simulink model "sixstep"  (R2017b)
settings: Solver=FixedStepDiscrete  StartTime=0.0  StopTime=10.0  FixedStep=0.003  RelTol=1e-3
libraries: simulink x1
settings Model: Creator=EW  LastModifiedBy=EW
settings DataIOCC: LimitDataPoints=on  SaveFormat=Array
settings OptimizationCC: LifeSpan=1
settings DebuggingCC: SFUnexpectedBacktrackingDiag=warning  SFNoUnconditionalDefaultTransitionDiag=warning  SFExecutionAtInitializationDiag=none
settings HardwareCC: ProdBitPerPointer=32  ProdBitPerSizeT=32  ProdBitPerPtrDiffT=32  ProdLargestAtomicInteger=Long  ProdLargestAtomicFloat=Double  ProdIntDivRoundTo=Undefined  ProdWordSize=32  ProdHWDeviceType=ARM Compatible->ARM Cortex
settings ModelReferenceCC: PropagateSignalLabelsOutOfModel=off
settings SFSimCC: MATLABDynamicMemAlloc=off
settings RTWCC: SystemTargetFile=mbed.tlc  TemplateMakefile=mbed.tmf  Description=Mbed Target (Embedded Target)  TargetLang=C++
settings CodeAppCC: IgnoreCustomStorageClasses=off  StateflowObjectComments=on
settings STFCustomTargetCC: TargetLibSuffix=.a  GenerateSampleERTMain=on  CombineOutputUpdateFcns=on  ERTCustomFileBanners=on  SupportContinuousTime=off  SupportNonInlinedSFcns=off  RemoveResetFunc=on  MATLABClassNameForMDSCustomization=Simulink.SoftwareTarget.ERTCustomization  ModelStepFunctionPrototypeControlCompliant=on  GRTInterface=off  SystemTargetFile=mbed.tlc
settings ERTTargetCC: MultiwordLength=2048  GenerateSampleERTMain=on  ParMdlRefBuildCompliant=off  CompOptLevelCompliant=off  ConcurrentExecutionCompliant=off  CPPClassGenCompliant=off  UseToolchainInfoCompliant=off  ERTCustomFileTemplate=mbed_file_process.tlc  ConvertIfToSwitch=off  SuppressUnreachableDefaultCases=off
settings ConfigComp: CovMetricSettings=dw  CovHtmlReporting=on  CovSaveCumulativeToWorkspaceVar=on  CovSaveSingleToWorkspaceVar=on  CovExternalEMLEnable=off

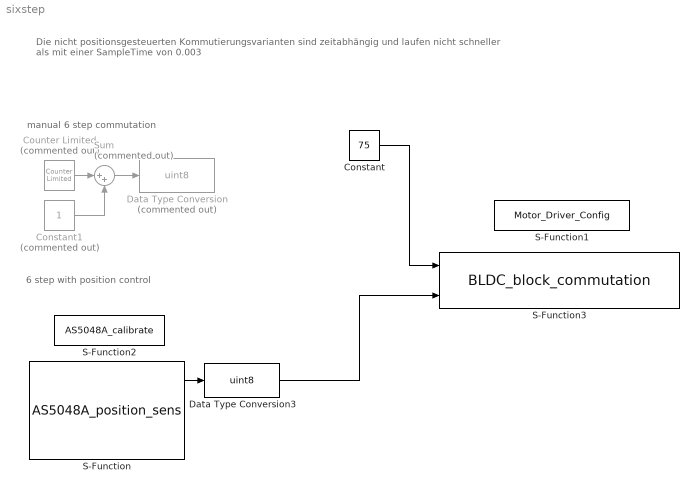
== system sixstep ==
  note: manual 6 step commutation
  note: 6 step with position control
  note: Die nicht positionsgesteuerten Kommutierungsvarianten sind zeitabhängig und laufen nicht schneller als mit einer SampleTime von 0.003
  Constant : Constant  Value=75  OutDataTypeStr=uint8
  Constant1 : Constant  Commented=on
  Counter Limited : simulink/Sources/Counter Limited  Commented=on  uplimit=5  tsamp=-1
  Data Type Conversion : DataTypeConversion  Commented=on  OutDataTypeStr=uint8
  Data Type Conversion3 : DataTypeConversion  OutDataTypeStr=uint8
  S-Function : S-Function  Priority=0  FunctionName=AS5048A_position_sens  Parameters=SampleTime, uint8(PortName), uint8(PinNumber)  SFunctionDeploymentMode=off  EnableBusSupport=off  mask{PortName=C, PinNumber=8, SampleTime=-1}
      mask prompts: PinNumber "Pin Number:"; SampleTime "Sample time (-1 for inherited)"
      mask TypeOptions PortName: A | B | C | D | F | G | H | I | J | K
      mask TypeOptions PinNumber: 0 | 1 | 2 | 3 | 4 | 5 | 6 | 7 | 8 | 9 | 10 | 11 | 12 | 13 | 14 | 15
      mask Display:
      | disp('AS5048')
      | port_label('output',1,'RAW');
      | port_label('output',2,'rad');
      | port_label('output',3,'rad/s');
  S-Function1 : S-Function  Priority=1  FunctionName=Motor_Driver_Config  Parameters=uint8(PWMUport),uint8(PWMVport),uint8(PWMWport),uint8(PWMUpin),uint8(PWMVpin),uint8(PWMWpin),uint8(EnableUport),uint8(EnableVport),uint8(EnableWport),uint8(EnableUpin),uint8(EnableVpin),uint8(EnableWpin)  SFunctionDeploymentMode=off  EnableBusSupport=off  mask{PWMUport=A, PWMUpin=8, PWMVport=A, PWMVpin=9, PWMWport=A, PWMWpin=10, EnableUport=C, EnableUpin=10, EnableVport=C, EnableVpin=11, EnableWport=C, EnableWpin=12}
      mask prompts: PWMUport "PWM   U:      Port Name"; PWMUpin "Pin Number"; PWMVport "PWM   V:      Port Name"; PWMVpin "Pin Number"; PWMWport "PWM  W:      Port Name"; PWMWpin "Pin Number"; EnableUport "Enable  U:     Port Name"; EnableUpin "Pin Number"; EnableVport "Enable  V:     Port Name"; EnableVpin "Pin Number"; EnableWport "Enable W:     Port Name"; EnableWpin "Pin Number"
      mask TypeOptions PWMUport: A | B | C | D | E | F | G | H | I | J
      mask TypeOptions PWMUpin: 0 | 1 | 2 | 3 | 4 | 5 | 6 | 7 | 8 | 9 | 10 | 11 | 12 | 13 | 14 | 15
      mask TypeOptions PWMVport: A | B | C | D | E | F | G | H | I | J
      mask TypeOptions PWMVpin: 0 | 1 | 2 | 3 | 4 | 5 | 6 | 7 | 8 | 9 | 10 | 11 | 12 | 13 | 14 | 15
      mask TypeOptions PWMWport: A | B | C | D | E | F | G | H | I | J
      mask TypeOptions PWMWpin: 0 | 1 | 2 | 3 | 4 | 5 | 6 | 7 | 8 | 9 | 10 | 11 | 12 | 13 | 14 | 15
      mask TypeOptions EnableUport: A | B | C | D | E | F | G | H | I | J
      mask TypeOptions EnableUpin: 0 | 1 | 2 | 3 | 4 | 5 | 6 | 7 | 8 | 9 | 10 | 11 | 12 | 13 | 14 | 15
      mask TypeOptions EnableVport: A | B | C | D | E | F | G | H | I | J
      mask TypeOptions EnableVpin: 0 | 1 | 2 | 3 | 4 | 5 | 6 | 7 | 8 | 9 | 10 | 11 | 12 | 13 | 14 | 15
      mask TypeOptions EnableWport: A | B | C | D | E | F | G | H | I | J
      mask TypeOptions EnableWpin: 0 | 1 | 2 | 3 | 4 | 5 | 6 | 7 | 8 | 9 | 10 | 11 | 12 | 13 | 14 | 15
  S-Function2 : S-Function  Priority=2  FunctionName=AS5048A_calibrate  SFunctionDeploymentMode=off  EnableBusSupport=off
      mask Display: disp('AS5048 calibration')
  S-Function3 : S-Function  Priority=3  FunctionName=BLDC_block_commutation  Parameters=SampleTime, uint8(power),uint8(mode)  SFunctionDeploymentMode=off  EnableBusSupport=off  mask{mode=Position controlled(AS5048A), power=on, SampleTime=-1}
      mask prompts: mode "chose operation mode"; power "Enable Power regulation port"; SampleTime "Sample time(-1 for inherited):"
      mask help:
      | power: is a pwm dutycycle in %   uses values 0-100
      |
      | step: provide the step sequence for the bldc driver uses values 1-6
      |
      | position: requires the position determined by the AS5048A_pos_sens Block
      mask TypeOptions mode: automatic steps | manual steps | Position controlled(AS5048A)
      mask Display:
      | disp(['6 Step Block Commutation'])
      | 
      | if power
      |     port_label('input',1,'power');
      | 
      |      if mode==2
      |         port_label('input',2,'step');
      |     end
      | 
      |     if mode==3
      |         port_label('input',2,'position');
      |     end
      | 
      | else
      |     if mode==2
      |         port_label('input',1,'step');
      |     end
      | 
      |     if mode==3
      |         port_label('input',1,'position');
      |     end
      | end
  Sum : Sum  Commented=on  Inputs=|++
  wires:
  S-Function/1 -> Data Type Conversion3/1
  Constant1/1 -> Sum/2
  Counter Limited/1 -> Sum/1
  Sum/1 -> Data Type Conversion/1
  Constant/1 -> S-Function3/1
  Data Type Conversion3/1 -> S-Function3/2
